simulink library "dgh_grc"  (R2024a)
settings: Solver=VariableStepAuto  StartTime=0.0  StopTime=10.0  RelTol=1e-3
undefined symbols (not defined in the file or in its folder): Diag1_iPhaCurrOverU_C, Diag1_iPhaCurrOverV_C, Diag1_iPhaCurrOverW_C, KDGH_bRstRteFault_flg, KDGH_FaultLevel2_flg_ovrdflg, KDGH_FaultLevel2_flg_ovrdval, KDGH_OverCurrent_A, KDGH_OverCurrent_flg_ovrdflg, KDGH_OverCurrent_flg_ovrdval, KDGH_OverCurrentErr_C, KDGH_OverCurrentHeal_C, KDGH_PhaCurrOverU_A, KDGH_PhaCurrOverV_A, KDGH_PhaCurrOverW_A, KDGH_RstPhaCurrOver_flg, KDGH_RstSumErr_flg, KDGH_SumErr_A, KDGH_SumErr_flg_ovrdflg, KDGH_SumErr_flg_ovrdval, KDGH_SumErrErr_C, KDGH_SumErrHeal_C, SampleTimeFOC, ZERO_FLOAT
libraries: GRC_Lib x13, simulink x4, Library x2
settings Model: Creator=FVT22063  LastModifiedBy=FVT22063

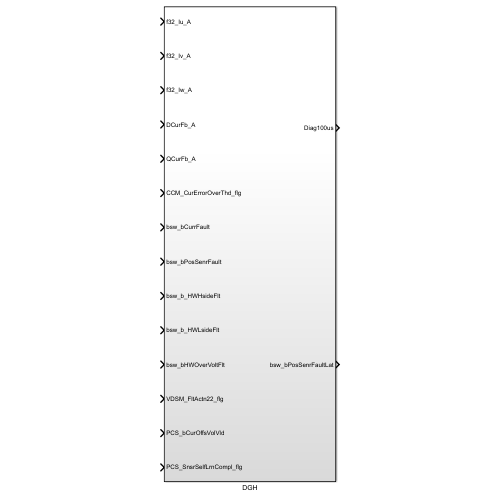
[thumbnail: Simulink's stored preview of the top-level diagram]
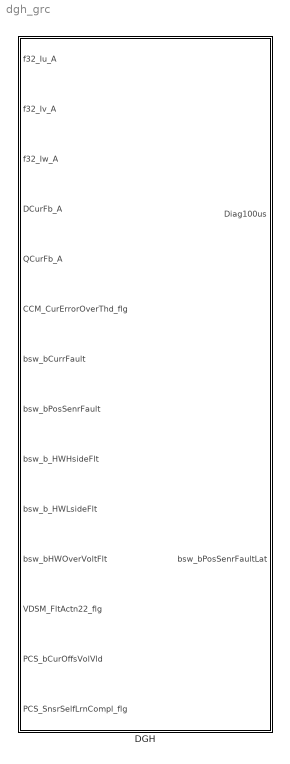
== system dgh_grc ==
  DGH : Subsystem

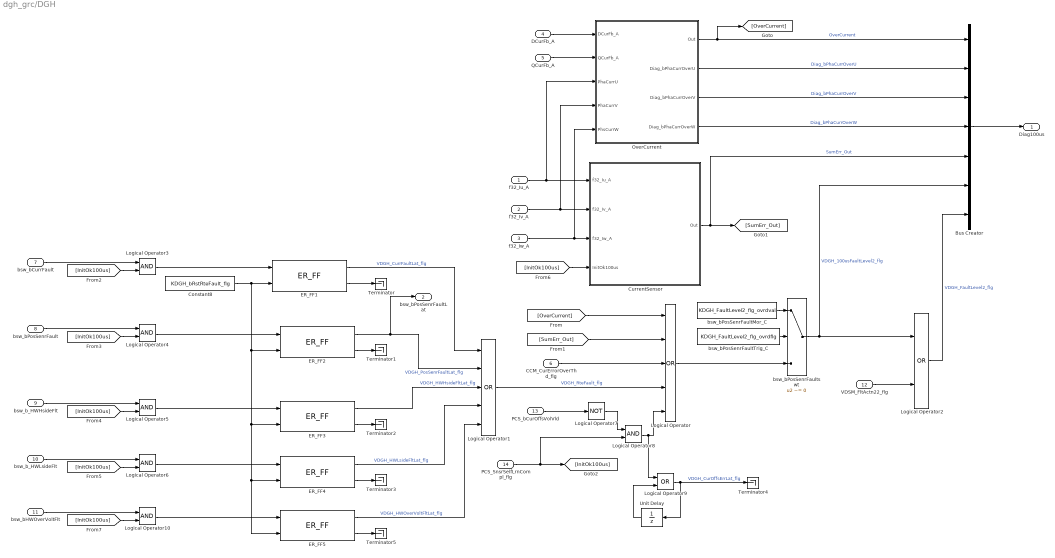
== system dgh_grc/DGH ==
  f32_Iu_A : Inport
  f32_Iv_A : Inport  Port=2
  f32_Iw_A : Inport  Port=3
  DCurFb_A : Inport  Port=4
  QCurFb_A : Inport  Port=5
  CCM_CurErrorOverThd_flg : Inport  Port=6  OutDataTypeStr=boolean
  bsw_bCurrFault : Inport  Port=7  OutDataTypeStr=boolean
  bsw_bPosSenrFault : Inport  Port=8  OutDataTypeStr=boolean
  bsw_b_HWHsideFlt : Inport  Port=9  OutDataTypeStr=boolean
  bsw_b_HWLsideFlt : Inport  Port=10  OutDataTypeStr=boolean
  bsw_bHWOverVoltFlt : Inport  Port=11  OutDataTypeStr=boolean
  VDSM_FltActn22_flg : Inport  Port=12  OutDataTypeStr=boolean
  PCS_bCurOffsVolVld : Inport  Port=13  OutDataTypeStr=boolean
  PCS_SnsrSelfLrnCompl_flg : Inport  Port=14  OutDataTypeStr=boolean
  Bus Creator : BusCreator  Inputs=7
  Constant8 : Constant  Value=KDGH_bRstRteFault_flg
  CurrentSensor : Subsystem  TreatAsAtomicUnit=on  RTWFcnName=CurrentSensor
      settings: RTWSystemCode=Nonreusable function  RTWFcnNameOpts=User specified
  ER_FF{1..5} (5 alike) : GRC_Lib/Memory/ER_FF  FalseVal=0  TrueVal=1
  Logical Operator : Logic  Operator=OR  Inputs=5  AllPortsSameDT=off  OutDataTypeStr=boolean
  Logical Operator1 : Logic  Operator=OR  Inputs=5  AllPortsSameDT=off  OutDataTypeStr=boolean
  Logical Operator{3..6,8,10} (6 alike) : Logic  AllPortsSameDT=off  OutDataTypeStr=boolean
  Logical Operator2 : Logic  Operator=OR  AllPortsSameDT=off  OutDataTypeStr=boolean
  Logical Operator7 : Logic  Operator=NOT  AllPortsSameDT=off  OutDataTypeStr=boolean
  Logical Operator9 : Logic  Operator=OR  AllPortsSameDT=off  OutDataTypeStr=boolean
  OverCurrent : Subsystem  TreatAsAtomicUnit=on  RTWFcnName=OverCurrent
      settings: RTWFcnNameOpts=User specified
  Terminator{,1..5} (6 alike) : Terminator
  Unit Delay : UnitDelay  SampleTime=-1  HasFrameUpgradeWarning=on
  bsw_bPosSenrFaultMor_C : Constant  Value=KDGH_FaultLevel2_flg_ovrdval
  bsw_bPosSenrFaultTrig_C : Constant  Value=KDGH_FaultLevel2_flg_ovrdflg
  bsw_bPosSenrFaultswt : Switch  Criteria=u2 ~= 0  SaturateOnIntegerOverflow=off  InputSameDT=off
  Diag100us : Outport  VectorParamsAs1DForOutWhenUnconnected=off
  bsw_bPosSenrFaultLat : Outport  Port=2  VectorParamsAs1DForOutWhenUnconnected=off
  wires:
  DCurFb_A/1 -> OverCurrent/1(DCurFb_A)
  QCurFb_A/1 -> OverCurrent/2(QCurFb_A)
  f32_Iu_A/1 -> OverCurrent/3(PhaCurrU), CurrentSensor/1(f32_Iu_A)
  f32_Iv_A/1 -> OverCurrent/4(PhaCurrV), CurrentSensor/2(f32_Iv_A)
  f32_Iw_A/1 -> OverCurrent/5(PhsCurrW), CurrentSensor/3(f32_Iw_A)
  Bus Creator/1 -> Diag100us/1
  CurrentSensor/1(Out) -> Bus Creator/5, [SumErr_Out]  "SumErr_Out"
  OverCurrent/1(Out) -> Bus Creator/1, [OverCurrent]  "OverCurrent"
  [OverCurrent] -> Logical Operator/1
  [SumErr_Out] -> Logical Operator/2
  bsw_bPosSenrFaultswt/1 -> Logical Operator2/1, Bus Creator/6  "VDGH_100usFaultLevel2_flg"
  OverCurrent/2(Diag_bPhaCurrOverU) -> Bus Creator/2  "Diag_bPhaCurrOverU"
  OverCurrent/3(Diag_bPhaCurrOverV) -> Bus Creator/3  "Diag_bPhaCurrOverV"
  OverCurrent/4(Diag_bPhaCurrOverW) -> Bus Creator/4  "Diag_bPhaCurrOverW"
  ER_FF1/1 -> Logical Operator1/1  "VDGH_CurrFaultLat_flg"
  Logical Operator1/1 -> Logical Operator/4  "VDGH_RteFault_flg"
  VDSM_FltActn22_flg/1 -> Logical Operator2/2
  Logical Operator2/1 -> Bus Creator/7  "VDGH_FaultLevel2_flg"
  CCM_CurErrorOverThd_flg/1 -> Logical Operator/3
  bsw_bPosSenrFaultMor_C/1 -> bsw_bPosSenrFaultswt/1
  bsw_bPosSenrFaultTrig_C/1 -> bsw_bPosSenrFaultswt/2
  Logical Operator/1 -> bsw_bPosSenrFaultswt/3
  PCS_SnsrSelfLrnCompl_flg/1 -> Logical Operator8/2, [InitOk100us]
  [InitOk100us] -> Logical Operator3/2
  [InitOk100us] -> Logical Operator4/2
  ER_FF2/1 -> bsw_bPosSenrFaultLat/1, Logical Operator1/2  "VDGH_PosSenrFaultLat_flg"
  ER_FF3/1 -> Logical Operator1/3  "VDGH_HWHsideFltLat_flg"
  [InitOk100us] -> Logical Operator5/2
  [InitOk100us] -> Logical Operator6/2
  Logical Operator6/1 -> ER_FF4/1
  PCS_bCurOffsVolVld/1 -> Logical Operator7/1
  Logical Operator7/1 -> Logical Operator8/1
  Logical Operator3/1 -> ER_FF1/1
  ER_FF1/2 -> Terminator/1
  Logical Operator4/1 -> ER_FF2/1
  ER_FF2/2 -> Terminator1/1
  Constant8/1 -> ER_FF5/2, ER_FF4/2, ER_FF3/2, ER_FF2/2, ER_FF1/2
  Logical Operator5/1 -> ER_FF3/1
  ER_FF3/2 -> Terminator2/1
  ER_FF4/1 -> Logical Operator1/4  "VDGH_HWLsideFltLat_flg"
  ER_FF4/2 -> Terminator3/1
  Logical Operator8/1 -> Logical Operator9/1, Logical Operator/5
  Logical Operator9/1 -> Terminator4/1, Unit Delay/1  "VDGH_CurOffsErrLat_flg"
  Unit Delay/1 -> Logical Operator9/2
  [InitOk100us] -> CurrentSensor/4(InitOk100us)
  bsw_bCurrFault/1 -> Logical Operator3/1
  bsw_bPosSenrFault/1 -> Logical Operator4/1
  bsw_b_HWHsideFlt/1 -> Logical Operator5/1
  bsw_b_HWLsideFlt/1 -> Logical Operator6/1
  bsw_bHWOverVoltFlt/1 -> Logical Operator10/1
  [InitOk100us] -> Logical Operator10/2
  ER_FF5/2 -> Terminator5/1
  ER_FF5/1 -> Logical Operator1/5  "VDGH_HWOverVoltFltLat_flg"
  Logical Operator10/1 -> ER_FF5/1

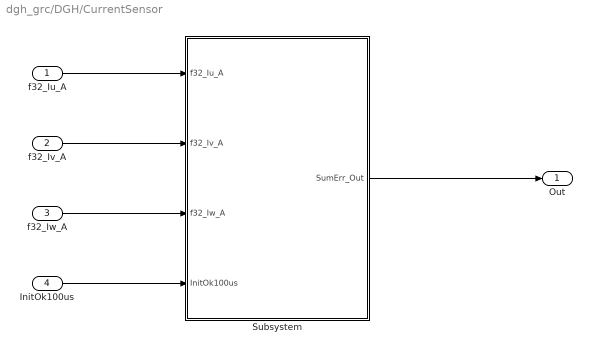
== system dgh_grc/DGH/CurrentSensor ==
  f32_Iu_A : Inport
  f32_Iv_A : Inport  Port=2
  f32_Iw_A : Inport  Port=3
  InitOk100us : Inport  Port=4  OutDataTypeStr=boolean
  Subsystem : Subsystem
  Out : Outport  VectorParamsAs1DForOutWhenUnconnected=off
  wires:
  Subsystem/1(SumErr_Out) -> Out/1
  f32_Iu_A/1 -> Subsystem/1(f32_Iu_A)
  f32_Iv_A/1 -> Subsystem/2(f32_Iv_A)
  f32_Iw_A/1 -> Subsystem/3(f32_Iw_A)
  InitOk100us/1 -> Subsystem/4(InitOk100us)

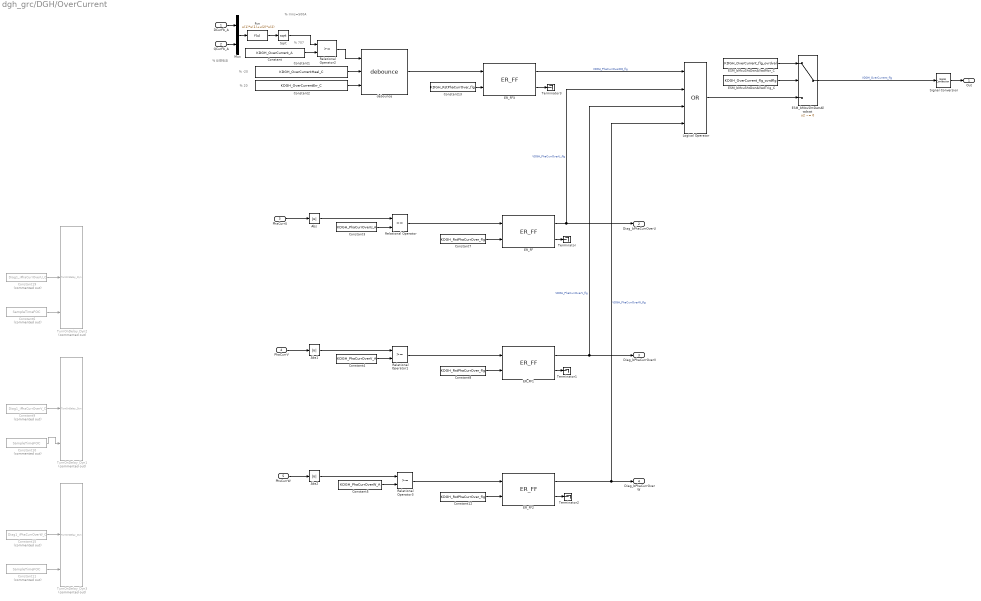
== system dgh_grc/DGH/OverCurrent ==
  note: % Irms=500A
  note: % 707
  note: % -20
  note: % 20
  note: % 反馈电流
  DCurFb_A : Inport
  QCurFb_A : Inport  Port=2
  PhaCurrU : Inport  Port=3
  PhaCurrV : Inport  Port=4
  PhsCurrW : Inport  Port=5
  Abs : Abs  SaturateOnIntegerOverflow=off
  Abs1 : Abs  SaturateOnIntegerOverflow=off
  Abs2 : Abs  SaturateOnIntegerOverflow=off
  Constant : Constant  Value=KDGH_OverCurrent_A  OutDataTypeStr=single
  Constant1 : Constant  Value=KDGH_OverCurrentHeal_C  OutDataTypeStr=int16
  Constant10 : Constant  Commented=on  Value=SampleTimeFOC
  Constant11 : Constant  Commented=on  Value=SampleTimeFOC
  Constant{7..8,12..13} (4 alike) : Constant  Value=KDGH_RstPhaCurrOver_flg
  Constant15 : Constant  Commented=on  Value=Diag1_iPhaCurrOverW_C
  Constant19 : Constant  Commented=on  Value=Diag1_iPhaCurrOverU_C
  Constant2 : Constant  Value=KDGH_OverCurrentErr_C  OutDataTypeStr=int16
  Constant3 : Constant  Value=KDGH_PhaCurrOverU_A
  Constant4 : Constant  Value=KDGH_PhaCurrOverV_A
  Constant5 : Constant  Value=KDGH_PhaCurrOverW_A
  Constant6 : Constant  Commented=on  Value=SampleTimeFOC
  Constant9 : Constant  Commented=on  Value=Diag1_iPhaCurrOverV_C
  ER_FF{,1..3} (4 alike) : GRC_Lib/Memory/ER_FF  FalseVal=0  TrueVal=1
  ESM_bMcuShtDwnAllwdMor_C : Constant  Value=KDGH_OverCurrent_flg_ovrdval
  ESM_bMcuShtDwnAllwdTrig_C : Constant  Value=KDGH_OverCurrent_flg_ovrdflg
  ESM_bMcuShtDwnAllwdswt : Switch  Criteria=u2 ~= 0  SaturateOnIntegerOverflow=off  InputSameDT=off
  Fcn : Fcn  Expr=u(1)*u(1)+u(2)*u(2)
  Logical Operator : Logic  Operator=OR  Inputs=4  AllPortsSameDT=off  OutDataTypeStr=boolean
  Mux : Mux  Inputs=2
  Relational Operator : RelationalOperator  OutDataTypeStr=boolean  RndMeth=Simplest  InputSameDT=off
  Relational Operator1 : RelationalOperator  OutDataTypeStr=boolean  RndMeth=Simplest  InputSameDT=off
  Relational Operator2 : RelationalOperator  OutDataTypeStr=boolean  InputSameDT=off
  Relational Operator3 : RelationalOperator  OutDataTypeStr=boolean  RndMeth=Simplest  InputSameDT=off
  Signal Conversion : SignalConversion  OverrideOpt=off
  Sqrt : Sqrt
  Terminator{,1..3} (4 alike) : Terminator
  TurnOnDelay_Dyn1 : GRC_Lib/Delay/TurnOnDelay_Dyn  Commented=on  IpDT=single
  TurnOnDelay_Dyn2 : GRC_Lib/Delay/TurnOnDelay_Dyn  Commented=on  IpDT=single
  TurnOnDelay_Dyn3 : GRC_Lib/Delay/TurnOnDelay_Dyn  Commented=on  IpDT=single
  debounce : Library/debounce  SystemSampleTime=-1  VariantActivationTime=update diagram  AllowFlexibleInterface=on  Latency=0  AutoFrameSizeCalculation=off
  Out : Outport  OutDataTypeStr=boolean  VectorParamsAs1DForOutWhenUnconnected=off
  Diag_bPhaCurrOverU : Outport  Port=2  OutDataTypeStr=boolean  VectorParamsAs1DForOutWhenUnconnected=off
  Diag_bPhaCurrOverV : Outport  Port=3  OutDataTypeStr=boolean  VectorParamsAs1DForOutWhenUnconnected=off
  Diag_bPhaCurrOverW : Outport  Port=4  OutDataTypeStr=boolean  VectorParamsAs1DForOutWhenUnconnected=off
  wires:
  Sqrt/1 -> Relational Operator2/1
  Constant2/1 -> debounce/3
  Constant/1 -> Relational Operator2/2
  ER_FF3/1 -> Logical Operator/1  "VDGH_PhaCurrOverDQ_flg"
  Relational Operator2/1 -> debounce/1
  Constant1/1 -> debounce/2
  Mux/1 -> Fcn/1
  QCurFb_A/1 -> Mux/2
  Fcn/1 -> Sqrt/1
  DCurFb_A/1 -> Mux/1
  PhaCurrU/1 -> Abs/1
  Constant3/1 -> Relational Operator/2
  PhaCurrV/1 -> Abs1/1
  Constant4/1 -> Relational Operator1/2
  PhsCurrW/1 -> Abs2/1
  Constant5/1 -> Relational Operator3/2
  ER_FF/1 -> Logical Operator/2, Diag_bPhaCurrOverU/1  "VDGH_PhaCurrOverU_flg"
  Relational Operator3/1 -> ER_FF2/1
  Relational Operator1/1 -> ER_FF1/1
  Relational Operator/1 -> ER_FF/1
  ESM_bMcuShtDwnAllwdswt/1 -> Signal Conversion/1  "VDGH_OverCurrent_flg"
  ESM_bMcuShtDwnAllwdTrig_C/1 -> ESM_bMcuShtDwnAllwdswt/2
  ESM_bMcuShtDwnAllwdMor_C/1 -> ESM_bMcuShtDwnAllwdswt/1
  Abs/1 -> Relational Operator/1
  Abs1/1 -> Relational Operator1/1
  Abs2/1 -> Relational Operator3/1
  Constant19/1 -> TurnOnDelay_Dyn2/2
  Constant6/1 -> TurnOnDelay_Dyn2/3
  Constant10/1 -> TurnOnDelay_Dyn1/3
  Constant9/1 -> TurnOnDelay_Dyn1/2
  Constant15/1 -> TurnOnDelay_Dyn3/2
  Constant11/1 -> TurnOnDelay_Dyn3/3
  ER_FF/2 -> Terminator/1
  Constant7/1 -> ER_FF/2
  Constant8/1 -> ER_FF1/2
  ER_FF1/2 -> Terminator1/1
  ER_FF1/1 -> Diag_bPhaCurrOverV/1, Logical Operator/3  "VDGH_PhaCurrOverV_flg"
  ER_FF2/1 -> Logical Operator/4, Diag_bPhaCurrOverW/1  "VDGH_PhaCurrOverW_flg"
  ER_FF2/2 -> Terminator2/1
  Constant12/1 -> ER_FF2/2
  Logical Operator/1 -> ESM_bMcuShtDwnAllwdswt/3
  Signal Conversion/1 -> Out/1
  Constant13/1 -> ER_FF3/2
  debounce/1 -> ER_FF3/1
  ER_FF3/2 -> Terminator3/1

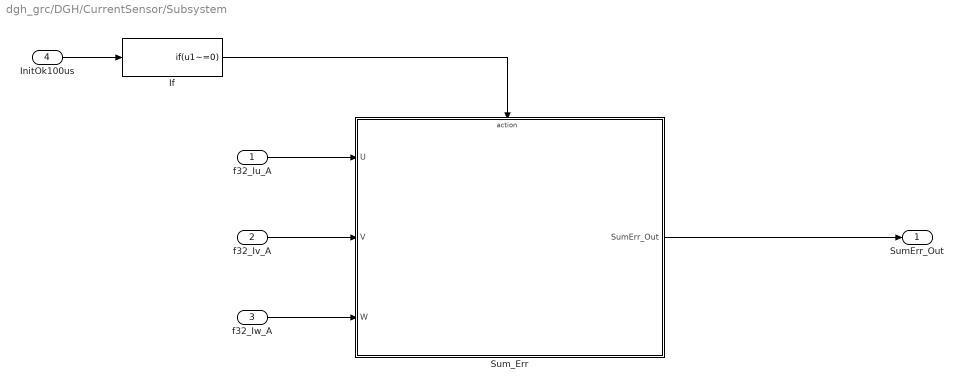
== system dgh_grc/DGH/CurrentSensor/Subsystem ==
  f32_Iu_A : Inport
  f32_Iv_A : Inport  Port=2
  f32_Iw_A : Inport  Port=3
  InitOk100us : Inport  Port=4  OutDataTypeStr=boolean
  If : If  IfExpression=u1~=0  ShowElse=off
  Sum_Err : Subsystem  TreatAsAtomicUnit=on
  SumErr_Out : Outport  VectorParamsAs1DForOutWhenUnconnected=off
  wires:
  Sum_Err/1(SumErr_Out) -> SumErr_Out/1
  f32_Iv_A/1 -> Sum_Err/2(V)
  f32_Iu_A/1 -> Sum_Err/1(U)
  f32_Iw_A/1 -> Sum_Err/3(W)
  InitOk100us/1 -> If/1
  If/1 -> Sum_Err/Action

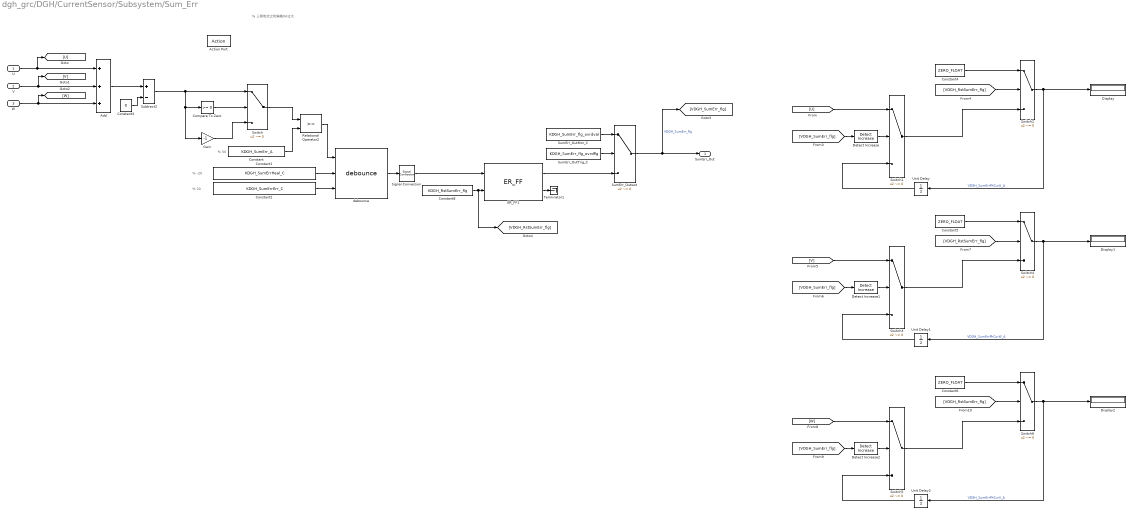
== system dgh_grc/DGH/CurrentSensor/Subsystem/Sum_Err ==
  note: % 50
  note: % 三相电流之和偏离0A过大
  note: % 20
  note: % -20
  U : Inport
  V : Inport  Port=2
  W : Inport  Port=3
  Action Port : ActionPort
  Add : Sum  Inputs=+++
  Compare To Zero : simulink/Logic and Bit Operations/Compare To Zero  relop=>=  OutDataTypeStr=boolean
  Constant : Constant  Value=KDGH_SumErr_A  OutDataTypeStr=single
  Constant1 : Constant  Value=KDGH_SumErrHeal_C  OutDataTypeStr=int16
  Constant2 : Constant  Value=KDGH_SumErrErr_C  OutDataTypeStr=int16
  Constant3 : Constant  Value=0  OutDataTypeStr=uint16
  Constant4 : Constant  Value=ZERO_FLOAT
  Constant5 : Constant  Value=ZERO_FLOAT
  Constant6 : Constant  Value=ZERO_FLOAT
  Constant8 : Constant  Value=KDGH_RstSumErr_flg
  Detect Increase : simulink/Logic and Bit Operations/Detect Increase  vinit=0.0  OutDataTypeStr=boolean
  Detect Increase1 : simulink/Logic and Bit Operations/Detect Increase  vinit=0.0  OutDataTypeStr=boolean
  Detect Increase2 : simulink/Logic and Bit Operations/Detect Increase  vinit=0.0  OutDataTypeStr=boolean
  Display : Display
  Display1 : Display
  Display2 : Display
  ER_FF1 : GRC_Lib/Memory/ER_FF  FalseVal=0  TrueVal=1
  Gain : Gain  Gain=-1  OutDataTypeStr=single
  Relational Operator2 : RelationalOperator  OutDataTypeStr=boolean  InputSameDT=off
  Signal Conversion : SignalConversion  OverrideOpt=off
  Subtract2 : Sum  Inputs=+-
  SumErr_OutMor_C : Constant  Value=KDGH_SumErr_flg_ovrdval
  SumErr_OutTrig_C : Constant  Value=KDGH_SumErr_flg_ovrdflg
  SumErr_Outswt : Switch  Criteria=u2 ~= 0  SaturateOnIntegerOverflow=off  InputSameDT=off
  Switch{,1..6} (7 alike) : Switch  Criteria=u2 ~= 0  SaturateOnIntegerOverflow=off  InputSameDT=off
  Terminator1 : Terminator
  Unit Delay : UnitDelay  SampleTime=-1  HasFrameUpgradeWarning=on
  Unit Delay1 : UnitDelay  SampleTime=-1  HasFrameUpgradeWarning=on
  Unit Delay2 : UnitDelay  SampleTime=-1  HasFrameUpgradeWarning=on
  debounce : Library/debounce  SystemSampleTime=-1  VariantActivationTime=update diagram  AllowFlexibleInterface=on  Latency=0  AutoFrameSizeCalculation=off
  SumErr_Out : Outport  VectorParamsAs1DForOutWhenUnconnected=off
  wires:
  Constant1/1 -> debounce/2
  Constant2/1 -> debounce/3
  Signal Conversion/1 -> ER_FF1/1
  debounce/1 -> Signal Conversion/1
  W/1 -> [W], Add/3
  V/1 -> [V], Add/2
  U/1 -> [U], Add/1
  Constant/1 -> Relational Operator2/2
  Relational Operator2/1 -> debounce/1
  Switch/1 -> Relational Operator2/1
  Constant3/1 -> Subtract2/2
  Add/1 -> Subtract2/1
  Gain/1 -> Switch/3
  Compare To Zero/1 -> Switch/2
  Subtract2/1 -> Switch/1, Compare To Zero/1, Gain/1
  SumErr_OutMor_C/1 -> SumErr_Outswt/1
  SumErr_OutTrig_C/1 -> SumErr_Outswt/2
  SumErr_Outswt/1 -> [VDGH_SumErr_flg], SumErr_Out/1  "VDGH_SumErr_flg"
  Constant8/1 -> [VDGH_RstSumErr_flg], ER_FF1/2
  ER_FF1/2 -> Terminator1/1
  ER_FF1/1 -> SumErr_Outswt/3
  [VDGH_SumErr_flg] -> Detect Increase/1
  [U] -> Switch1/1
  Unit Delay/1 -> Switch1/3
  Detect Increase/1 -> Switch1/2
  [VDGH_RstSumErr_flg] -> Switch2/2
  Constant4/1 -> Switch2/1
  Switch1/1 -> Switch2/3
  Switch2/1 -> Unit Delay/1, Display/1  "VDGH_SumErrPhCurU_A"
  Switch3/1 -> Switch4/3
  [V] -> Switch3/1
  Unit Delay1/1 -> Switch3/3
  Constant5/1 -> Switch4/1
  Detect Increase1/1 -> Switch3/2
  [VDGH_RstSumErr_flg] -> Switch4/2
  Switch4/1 -> Unit Delay1/1, Display1/1  "VDGH_SumErrPhCurW_A"
  [VDGH_SumErr_flg] -> Detect Increase1/1
  Switch5/1 -> Switch6/3
  [W] -> Switch5/1
  Unit Delay2/1 -> Switch5/3
  Constant6/1 -> Switch6/1
  Detect Increase2/1 -> Switch5/2
  [VDGH_RstSumErr_flg] -> Switch6/2
  Switch6/1 -> Unit Delay2/1, Display2/1  "VDGH_SumErrPhCurV_A"
  [VDGH_SumErr_flg] -> Detect Increase2/1
